simulink model "Efficiency_Map_ID_Validation_Sim"  (R2017b)
settings: Solver=VariableStepAuto  StartTime=0.0  StopTime=10.0  RelTol=1e-3
values from neighbouring files (symbols this model uses):
  motor_speed = mtr_speed_rad(j)    [Efficiency_Map_Validation.m]
  motor_torque = mtr_torque(i)    [Efficiency_Map_Validation.m]
  p00 = -215.8    [Efficiency_Map_Validation.m]    (also in Efficiency_Maps.m)
  p01 = 3.368    [Efficiency_Map_Validation.m]    (also in Efficiency_Maps.m)
  p02 = -0.0178    [Efficiency_Map_Validation.m]    (also in Efficiency_Maps.m)
  p03 = 6.515e-05    [Efficiency_Map_Validation.m]    (also in Efficiency_Maps.m)
  p10 = 4.164    [Efficiency_Map_Validation.m]    (also in Efficiency_Maps.m)
  p11 = 0.04408    [Efficiency_Map_Validation.m]    (also in Efficiency_Maps.m)
  p12 = 9.874e-05    [Efficiency_Map_Validation.m]    (also in Efficiency_Maps.m)
  p20 = -0.009417    [Efficiency_Map_Validation.m]    (also in Efficiency_Maps.m)
  p21 = 5.981e-06    [Efficiency_Map_Validation.m]    (also in Efficiency_Maps.m)
  p30 = 5.161e-06    [Efficiency_Map_Validation.m]    (also in Efficiency_Maps.m)
settings Model: Creator=Robert Wygant  LastModifiedBy=Robert Wygant

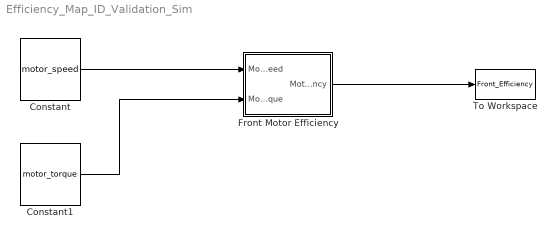
== system Efficiency_Map_ID_Validation_Sim ==
  Constant : Constant  Value=motor_speed
  Constant1 : Constant  Value=motor_torque
  Front Motor Efficiency : Subsystem
      mask Display:
      | color('green')
      | disp("Motor Efficiency")
  To Workspace : ToWorkspace  VariableName=Front_Efficiency  SampleTime=-1
      settings: MaxDataPoints=1  Save2DSignal=2-D array (concatenate along first dimension)
  wires:
  Constant/1 -> Front Motor Efficiency/1(Motor_speed)
  Constant1/1 -> Front Motor Efficiency/2(Motor_torque)
  Front Motor Efficiency/1(Motor_efficiency) -> To Workspace/1

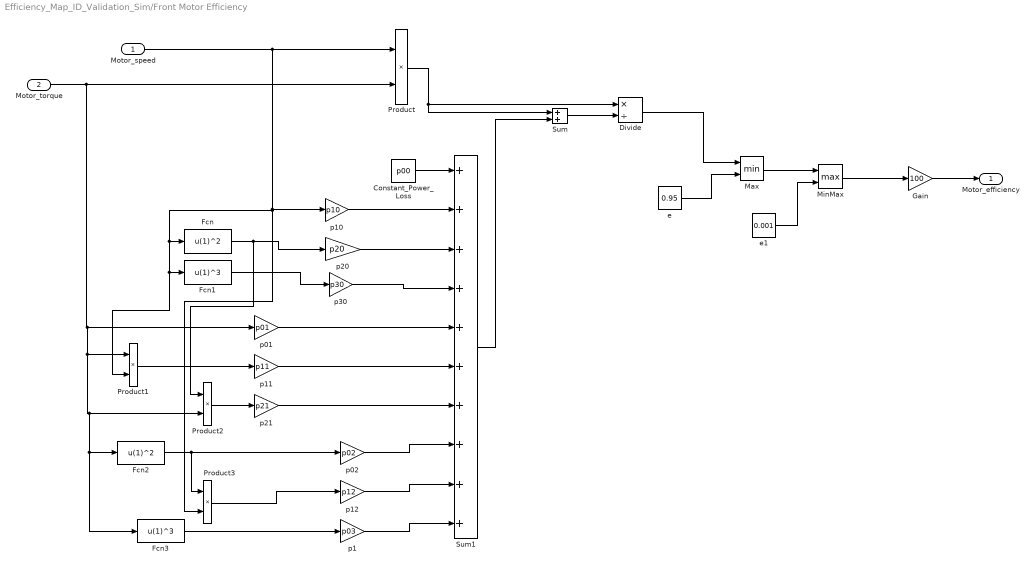
== system Efficiency_Map_ID_Validation_Sim/Front Motor Efficiency ==
  Motor_speed : Inport
  Motor_torque : Inport  Port=2
  Constant_Power_Loss : Constant  Value=p00
  Divide : Product  Inputs=*/
  Fcn : Fcn  Expr=u(1)^2
  Fcn1 : Fcn  Expr=u(1)^3
  Fcn2 : Fcn  Expr=u(1)^2
  Fcn3 : Fcn  Expr=u(1)^3
  Gain : Gain  Gain=100
  Max : MinMax  Inputs=2
  MinMax : MinMax  Function=max  Inputs=2
  Product{,1..3} (4 alike) : Product
  Sum : Sum
  Sum1 : Sum  Inputs=++++++++++
  e : Constant  Value=0.95
  e1 : Constant  Value=0.001
  p01 : Gain  Gain=p01
  p02 : Gain  Gain=p02
  p1 : Gain  Gain=p03
  p10 : Gain  Gain=p10
  p11 : Gain  Gain=p11
  p12 : Gain  Gain=p12
  p20 : Gain  Gain=p20
  p21 : Gain  Gain=p21
  p30 : Gain  Gain=p30
  Motor_efficiency : Outport
  wires:
  Max/1 -> MinMax/1
  e/1 -> Max/2
  Fcn3/1 -> p1/1
  p1/1 -> Sum1/10
  p12/1 -> Sum1/9
  Product3/1 -> p12/1
  Motor_torque/1 -> Product/2, p01/1, Product1/1, Product2/2, Fcn2/1, Fcn3/1
  p01/1 -> Sum1/5
  p11/1 -> Sum1/6
  p21/1 -> Sum1/7
  p02/1 -> Sum1/8
  Fcn2/1 -> p02/1, Product3/1
  Product2/1 -> p21/1
  Product1/1 -> p11/1
  p30/1 -> Sum1/4
  Fcn1/1 -> p30/1
  Fcn/1 -> p20/1, Product2/1
  p20/1 -> Sum1/3
  p10/1 -> Sum1/2
  Constant_Power_Loss/1 -> Sum1/1
  Motor_speed/1 -> Product/1, p10/1, Fcn/1, Fcn1/1, Product1/2, Product3/2
  Divide/1 -> Max/1
  Sum1/1 -> Sum/2
  Sum/1 -> Divide/2
  Product/1 -> Divide/1, Sum/1
  MinMax/1 -> Gain/1
  e1/1 -> MinMax/2
  Gain/1 -> Motor_efficiency/1
